simulink model "working_4states2"  (R2022b)
settings: Solver=FixedStepAuto  StartTime=0.0  StopTime=10.0  FixedStep=1e-3  RelTol=1e-3  EnableMultiTasking=on
undefined symbols (not defined in the file): a, A0, A1, b, c, D0, D1, D10, D11, D12, D13, D2, D3, D4, D5, D6, D7, D8, D9, PTA0, PTA1, PTA2, PTB2, PTB23, PTB3, PTB9, PTC16, PTC17, PTC2, PTC3, PTC4, PTD0, PTD1, PTD2, PTD3
libraries: frdmk64flib x22, etargetslib x2, dspstat3 x1, hdlsllib x1
settings Model: ExtModeTrigDuration=5  Creator=qasim  LastModifiedBy=Venka
settings SolverCC: AlgebraicLoopSolver=TrustRegion
settings OptimizationCC: EnhancedBackFolding=on  PassReuseOutputArgsAs=Individual arguments  ZeroExternalMemoryAtStartup=off  ZeroInternalMemoryAtStartup=off  MaxStackSize=64  OptimizeBlockOrder=speed  DifferentSizesBufferReuse=on  OptimizationCustomize=off  EfficientTunableParamExpr=on
settings DebuggingCC: ParameterTunabilityLossMsg=error  UnconnectedInputMsg=warning  UnconnectedOutputMsg=warning  UnconnectedLineMsg=warning  SFMachineParentedDataDiag=warning
settings HardwareCC: ProdBitPerPointer=32  ProdBitPerSizeT=32  ProdBitPerPtrDiffT=32  ProdLargestAtomicInteger=Long  ProdLargestAtomicFloat=Double  ProdWordSize=32  ProdHWDeviceType=ARM Compatible->ARM Cortex
settings ModelReferenceCC: EnableRefExpFcnMdlSchedulingChecks=on
settings SFSimCC: MATLABDynamicMemAlloc=off
settings RTWCC: Description=Embedded Coder  SystemTargetFile=ert.tlc  HardwareBoard=NXP FRDM-K64F  TLCOptions="-aInlineSetEventsForThisBaseRateFcn=TLC_FALSE -aSuppressMultiTaskScheduler=TLC_FALSE  -aRateBasedStepFcn=0"  TemplateMakefile=ert_default_tmf  Toolchain=GNU Tools for ARM Embedded Processors
settings CodeAppCC: ForceParamTrailComments=on  IgnoreCustomStorageClasses=off  OperatorAnnotations=on  SimulinkDataObjDesc=on  SFDataObjDesc=on  InsertBlockDesc=on

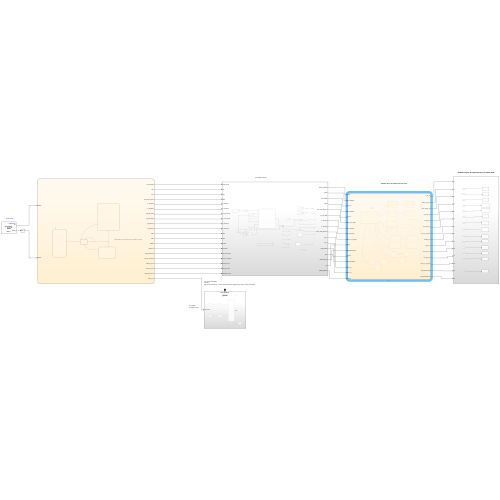
[thumbnail: Simulink's stored preview of the top-level diagram]
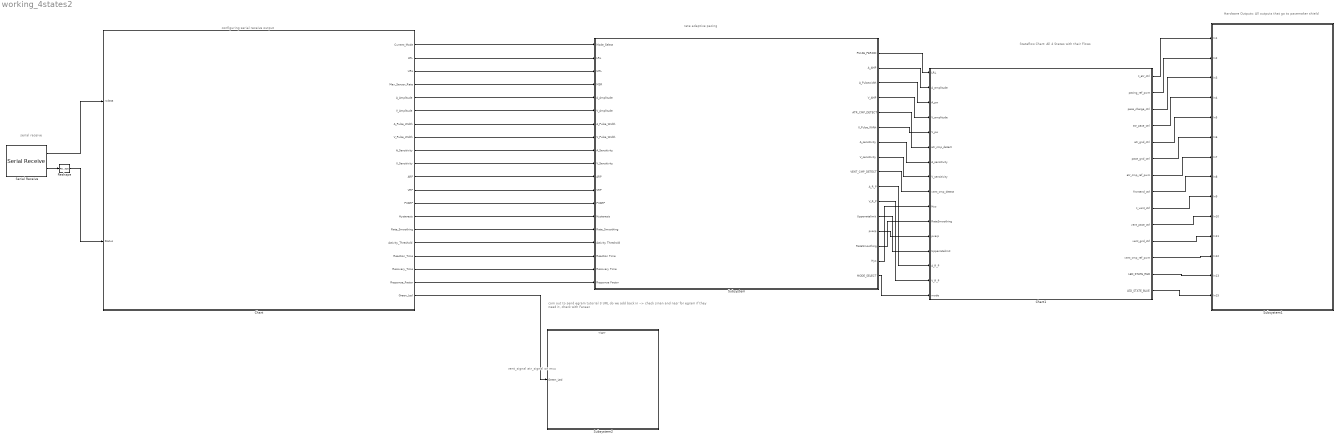
== system working_4states2 ==
  note: vent_signal
      | atr_signal on mcu
  note: rate adaptive pacing
  note: com out to send egram
      | tutorial 3
      | URL do we add back in --> check sinan and nasr for egram if they need it, check with Faraaz
  note: configuring serial receive output
  note: serial receive
  note: Stateflow Chart: All 4 States with their Flows
  note: Hardware Outputs: All outputs that go to pacemaker shield
  Chart : Stateflow chart  TreatAsAtomicUnit=on
      settings: PortSchema="{\"entries\":[{\"content\":{\"sides\":[{\"content\":{\"connectorIds\":[\"In1\",\"In2\"]},\"type\":\"ConnectorPlacement.EquallySpacedRectSide\",\"uuid\":\"8252b096-ee07-43c1-a389-abcea636169e\"},{\"content\":{\"connectorIds\":[\"Out12\",\"Out1\",\"Out16\",\"Out6\",\"Out8\",\"Out18\",\"Out10\",\"Out2\",\"Out11\",\"Out19\",\"Out9\",\"Out17\",\"Out14\",\"Out13\",\"Out15\",\"Out7\",\"Out5\",\"Out4\",\"Out3\",\"Out20\"],\"side\":\"RIGHT\"},\"type\":\"ConnectorPlacement.EquallySpacedRectSide\",\"uuid\":\"6509d00a-23de-4c51-a2fd-aafeb9bf7496\"},{\"content\":{\"connectorIds\":[],\"side\":\"TOP\"},\"type\":\"ConnectorPlacement.EquallySpacedRectSide\",\"uuid\":\"7ce604d1-90fd-4e3f-a76f-dae8bfc557ef\"}]},\"type\":\"ConnectorPlacement.EquallySpacedConnector\",\"uuid\":\"aa5568fb-1845-4bf2-8442-67645cd91be1\"}],\"packageUris\":[\"http://schema.mathworks.com/mf0/Connector/19700101\"],\"version\":\"1.0\"}"
  Chart1 : Stateflow chart  TreatAsAtomicUnit=on
      settings: PortSchema="{\"entries\":[{\"content\":{\"sides\":[{\"content\":{\"connectorIds\":[\"In1\",\"In4\",\"In5\",\"In9\",\"In10\",\"In2\",\"In7\",\"In8\",\"In6\",\"In11\",\"In12\",\"In13\",\"In14\",\"In15\",\"In16\",\"In3\"]},\"type\":\"ConnectorPlacement.EquallySpacedRectSide\",\"uuid\":\"9ebc7a7a-d83d-48fa-a96d-77ac692b9900\"},{\"content\":{\"connectorIds\":[\"Out1\",\"Out2\",\"Out3\",\"Out4\",\"Out5\",\"Out6\",\"Out7\",\"Out8\",\"Out9\",\"Out10\",\"Out11\",\"Out12\",\"Out13\",\"Out14\"],\"side\":\"RIGHT\"},\"type\":\"ConnectorPlacement.EquallySpacedRectSide\",\"uuid\":\"b238fc19-89ba-47ab-b52b-92ee760fd465\"},{\"content\":{\"connectorIds\":[],\"side\":\"TOP\"},\"type\":\"ConnectorPlacement.EquallySpacedRectSide\",\"uuid\":\"260cfadc-f762-444a-84c6-2a5806da8ce4\"}]},\"type\":\"ConnectorPlacement.EquallySpacedConnector\",\"uuid\":\"de40cf96-4d97-4a60-8c1b-853002d7031e\"}],\"packageUris\":[\"http://schema.mathworks.com/mf0/Connector/19700101\"],\"version\":\"1.0\"}"
  Reshape : Reshape
  Serial Receive : frdmk64flib/Serial Receive  SCIModule=0  Baudrate=uint32(9600)  Parity=None  StopBits=1  HardwareFlowControl=None  ByteOrder=LittleEndian  DataType=uint8  DataLength=52  BlockingMode=off  OutputStatus=on  SampleTime=-1
  Subsystem : Subsystem
  Subsystem1 : Subsystem
  Subsystem2 : Subsystem
  wires:
  Chart1/7(atr_cmp_ref_pwm) -> Subsystem1/7(In7)
  Chart1/5(atr_gnd_ctrl) -> Subsystem1/5(In5)
  Chart1/2(pacing_ref_pwm) -> Subsystem1/2(In2)
  Chart1/8(frontend_ctrl) -> Subsystem1/8(In8)
  Chart1/13(LED_STATE_RED) -> Subsystem1/13(In13)
  Chart1/3(pace_charge_ctrl) -> Subsystem1/3(In3)
  Chart1/11(vent_gnd_ctrl) -> Subsystem1/11(In11)
  Chart1/4(atr_pace_ctrl) -> Subsystem1/4(In4)
  Chart1/12(vent_cmp_ref_pwm) -> Subsystem1/12(In12)
  Chart1/9(z_vent_ctrl) -> Subsystem1/9(In9)
  Chart1/14(LED_STATE_BLUE) -> Subsystem1/14(In15)
  Chart1/1(z_atr_ctrl) -> Subsystem1/1(In1)
  Chart1/10(vent_pace_ctrl) -> Subsystem1/10(In10)
  Chart1/6(pace_gnd_ctrl) -> Subsystem1/6(In6)
  Subsystem/5(ATR_CMP_DETECT) -> Chart1/2(atr_cmp_detect)
  Subsystem/9(VENT_CMP_DETECT) -> Chart1/6(vent_cmp_detect)
  Subsystem/16(MODE_SELECT) -> Chart1/3(mode)
  Subsystem/2(A_AMP) -> Chart1/4(A_amplitude)
  Subsystem/3(A_Pulsewidth) -> Chart1/5(A_pw)
  Subsystem/1(PULSE_PERIOD) -> Chart1/1(LRL)
  Serial Receive/1 -> Chart/1(rxdata)
  Chart/1(LRL) -> Subsystem/2(LRL)
  Chart/6(Max_Sensor_Rate) -> Subsystem/4(MSR)
  Chart/7(Activity_Threshold) -> Subsystem/16(Activity Threshold)
  Chart/3(Response_Factor) -> Subsystem/19(Response Factor)
  Chart/5(Reaction_Time) -> Subsystem/17(Reaction Time)
  Chart/4(Recovery_Time) -> Subsystem/18(Recovery Time)
  Chart/8(A_Amplitude) -> Subsystem/5(A_Amplitude)
  Chart/11(A_Sensitivity) -> Subsystem/9(A_Sensitivity)
  Chart/19(V_Sensitivity) -> Subsystem/10(V_Sensitivity)
  Chart/18(V_Amplitude) -> Subsystem/6(V_Amplitude)
  Chart/10(A_Pulse_Width) -> Subsystem/7(A_Pulse_Width)
  Chart/2(V_Pulse_Width) -> Subsystem/8(V_Pulse_Width)
  Chart/9(ARP) -> Subsystem/11(ARP)
  Chart/12(Current_Mode) -> Subsystem/1(Mode_Select)
  Chart/13(Hysteresis) -> Subsystem/14(Hysteresis)
  Chart/17(VRP) -> Subsystem/12(VRP)
  Chart/16(URL) -> Subsystem/3(URL)
  Chart/14(PVARP) -> Subsystem/13(PVARP)
  Chart/15(Rate_Smoothing) -> Subsystem/15(Rate_Smoothing)
  Subsystem/4(V_AMP) -> Chart1/9(V_amplitude)
  Subsystem/6(V_Pulse_Wifth) -> Chart1/10(V_pw)
  Subsystem/7(A_sensitivity) -> Chart1/7(A_sensitivity)
  Subsystem/8(V_sensitivity) -> Chart1/8(V_sensitivity)
  Subsystem/15(Hys) -> Chart1/11(Hys)
  Subsystem/14(RateSmoothing) -> Chart1/12(RateSmoothing)
  Subsystem/13(pvarp) -> Chart1/13(pvarp)
  Subsystem/12(Upperratelimit) -> Chart1/14(Upperratelimit)
  Subsystem/11(V_R_P) -> Chart1/16(V_R_P)
  Subsystem/10(A_R_P) -> Chart1/15(A_R_P)
  Serial Receive/2 -> Reshape/1
  Reshape/1 -> Chart/2(Status)
  Chart/20(Green_Led) -> Subsystem2/1(Green_Led)

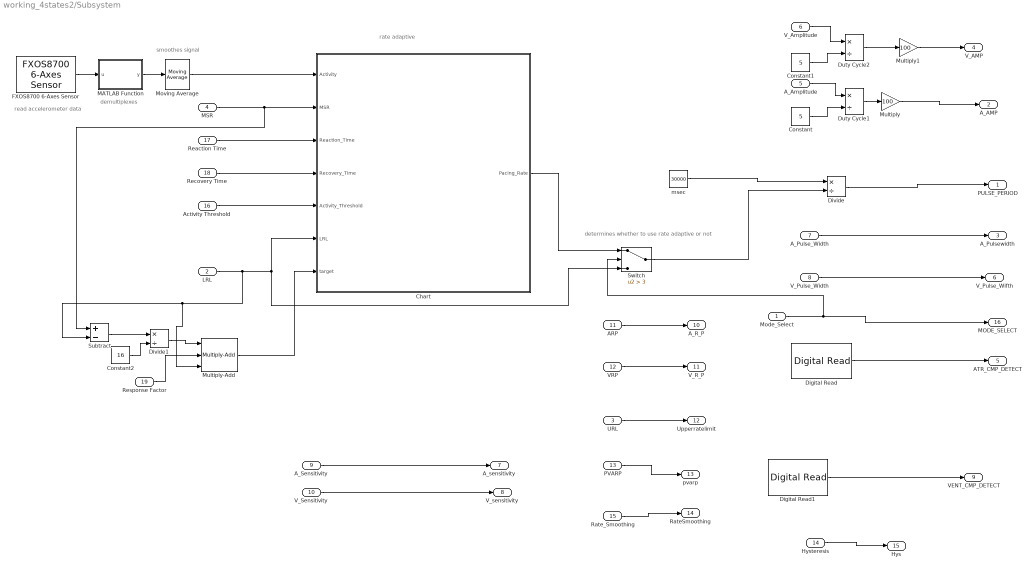
== system working_4states2/Subsystem ==
  note: rate adaptive
  note: determines whether to use rate adaptive or not
  note: smoothes signal
  note: demultiplexes
  note: read accelerometer data
  Mode_Select : Inport
  LRL : Inport  Port=2
  URL : Inport  Port=3
  MSR : Inport  Port=4
  A_Amplitude : Inport  Port=5
  V_Amplitude : Inport  Port=6
  A_Pulse_Width : Inport  Port=7
  V_Pulse_Width : Inport  Port=8
  A_Sensitivity : Inport  Port=9
  V_Sensitivity : Inport  Port=10
  ARP : Inport  Port=11
  VRP : Inport  Port=12
  PVARP : Inport  Port=13
  Hysteresis : Inport  Port=14
  Rate_Smoothing : Inport  Port=15
  Activity Threshold : Inport  Port=16
  Reaction Time : Inport  Port=17
  Recovery Time : Inport  Port=18
  Response Factor : Inport  Port=19
  Chart : Stateflow chart  TreatAsAtomicUnit=on
  Constant : Constant  Value=5
  Constant1 : Constant  Value=5
  Constant2 : Constant  Value=16
  Digital Read : frdmk64flib/Digital Read  Whichpin=PTC16 (D0)  SampleTime=-1
  Digital Read1 : frdmk64flib/Digital Read  Whichpin=PTC17 (D1)  SampleTime=-1
  Divide : Product  Inputs=*/
  Divide1 : Product  Inputs=*/
  Duty Cycle1 : Product  Inputs=*/
  Duty Cycle2 : Product  Inputs=*/
  FXOS8700 6-Axes Sensor : frdmk64flib/FXOS8700 6-Axes Sensor  Activesensor=Accelerometer only  ODR=100Hz  HybridODR=400Hz  Accelfullrange=-4g to +4g  SampleTime=-1
  MATLAB Function : MATLAB Function  TreatAsAtomicUnit=on
  Moving Average : dspstat3/Moving Average  Method=Sliding window  ForgettingFactorPort=off  SpecifyWindowLength=on  WindowLength=500  OverlapLength=499  AllowArbitraryInputLength=off  ForgettingFactor=0.9  SimulateUsing=Code generation
  Multiply : Gain  Gain=100
  Multiply-Add : hdlsllib/HDL Operations/Multiply-Add  Function=c+(a.*b)  datatype=Inherit: Inherit via internal rule  DoSatur=off  FMA=off
  Multiply1 : Gain  Gain=100
  Subtract : Sum  Inputs=+-
  Switch : Switch  Criteria=u2 > Threshold  Threshold=3  SaturateOnIntegerOverflow=off  InputSameDT=off
  msec : Constant  Value=30000
  PULSE_PERIOD : Outport
  A_AMP : Outport  Port=2
  A_Pulsewidth : Outport  Port=3
  V_AMP : Outport  Port=4
  ATR_CMP_DETECT : Outport  Port=5
  V_Pulse_Wifth : Outport  Port=6
  A_sensitivity : Outport  Port=7
  V_sensitivity : Outport  Port=8
  VENT_CMP_DETECT : Outport  Port=9
  A_R_P : Outport  Port=10
  V_R_P : Outport  Port=11
  Upperratelimit : Outport  Port=12
  pvarp : Outport  Port=13
  RateSmoothing : Outport  Port=14
  Hys : Outport  Port=15
  MODE_SELECT : Outport  Port=16
  wires:
  Moving Average/1 -> Chart/1(Activity)
  LRL/1 -> Multiply-Add/3, Subtract/2, Switch/3, Chart/6(LRL)
  Response Factor/1 -> Multiply-Add/2
  FXOS8700 6-Axes Sensor/1 -> MATLAB Function/1(u)
  Activity Threshold/1 -> Chart/5(Activity_Threshold)
  MSR/1 -> Subtract/1, Chart/2(MSR)
  Reaction Time/1 -> Chart/3(Reaction_Time)
  MATLAB Function/1(y) -> Moving Average/1
  Chart/1(Pacing_Rate) -> Switch/1
  Recovery Time/1 -> Chart/4(Recovery_Time)
  Multiply/1 -> A_AMP/1
  A_Amplitude/1 -> Duty Cycle1/1
  Duty Cycle1/1 -> Multiply/1
  Divide/1 -> PULSE_PERIOD/1
  Mode_Select/1 -> Switch/2, MODE_SELECT/1
  Constant/1 -> Duty Cycle1/2
  msec/1 -> Divide/1
  Digital Read/1 -> ATR_CMP_DETECT/1
  Digital Read1/1 -> VENT_CMP_DETECT/1
  Constant1/1 -> Duty Cycle2/2
  V_Amplitude/1 -> Duty Cycle2/1
  Duty Cycle2/1 -> Multiply1/1
  Multiply1/1 -> V_AMP/1
  ARP/1 -> A_R_P/1
  VRP/1 -> V_R_P/1
  URL/1 -> Upperratelimit/1
  PVARP/1 -> pvarp/1
  Rate_Smoothing/1 -> RateSmoothing/1
  Hysteresis/1 -> Hys/1
  Subtract/1 -> Divide1/1
  Divide1/1 -> Multiply-Add/1
  Constant2/1 -> Divide1/2
  Multiply-Add/1 -> Chart/7(target)
  A_Sensitivity/1 -> A_sensitivity/1
  V_Sensitivity/1 -> V_sensitivity/1
  Switch/1 -> Divide/2
  A_Pulse_Width/1 -> A_Pulsewidth/1
  V_Pulse_Width/1 -> V_Pulse_Wifth/1

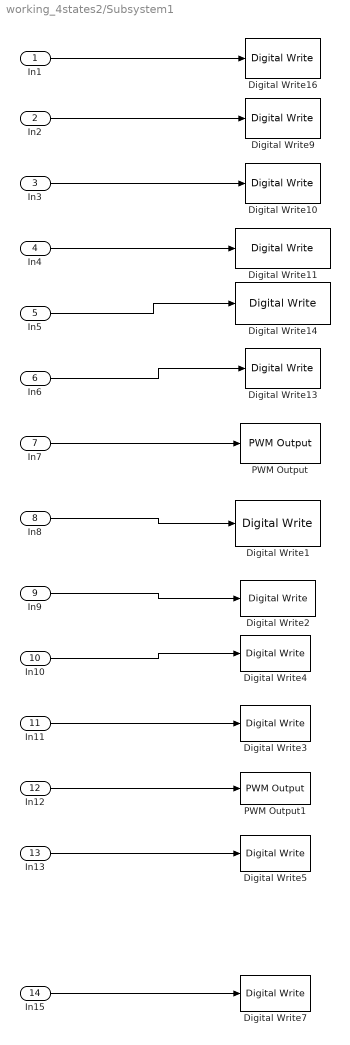
== system working_4states2/Subsystem1 ==
  In1 : Inport
  In2 : Inport  Port=2
  In3 : Inport  Port=3
  In4 : Inport  Port=4
  In5 : Inport  Port=5
  In6 : Inport  Port=6
  In7 : Inport  Port=7
  In8 : Inport  Port=8
  In9 : Inport  Port=9
  In10 : Inport  Port=10
  In11 : Inport  Port=11
  In12 : Inport  Port=12
  In13 : Inport  Port=13
  In15 : Inport  Port=14
  Digital Write1 : frdmk64flib/Digital Write  Whichpin=PTD1 (D13)
  Digital Write10 : frdmk64flib/Digital Write  Whichpin=PTB9 (D2)
  Digital Write11 : frdmk64flib/Digital Write  Whichpin=PTA0 (D8)
  Digital Write13 : frdmk64flib/Digital Write  Whichpin=PTD0 (D10)
  Digital Write14 : frdmk64flib/Digital Write  Whichpin=PTD2 (D11)
  Digital Write16 : frdmk64flib/Digital Write  Whichpin=PTB23 (D4)
  Digital Write2 : frdmk64flib/Digital Write  Whichpin=PTC3 (D7)
  Digital Write3 : frdmk64flib/Digital Write  Whichpin=PTD3 (D12)
  Digital Write4 : frdmk64flib/Digital Write  Whichpin=PTC4 (D9)
  Digital Write5 : frdmk64flib/Digital Write  Whichpin=RED_LED
  Digital Write7 : frdmk64flib/Digital Write  Whichpin=BLUE_LED
  Digital Write9 : frdmk64flib/Digital Write  Whichpin=PTA2 (D5)
  PWM Output : frdmk64flib/PWM Output  Whichpin=PTC2 (D6)  InitialFrequency=2000  InitialDutyCycle=0
  PWM Output1 : frdmk64flib/PWM Output  Whichpin=PTA1 (D3)  InitialFrequency=2000  InitialDutyCycle=0
  wires:
  In1/1 -> Digital Write16/1
  In2/1 -> Digital Write9/1
  In3/1 -> Digital Write10/1
  In4/1 -> Digital Write11/1
  In5/1 -> Digital Write14/1
  In6/1 -> Digital Write13/1
  In7/1 -> PWM Output/1
  In8/1 -> Digital Write1/1
  In9/1 -> Digital Write2/1
  In10/1 -> Digital Write4/1
  In11/1 -> Digital Write3/1
  In12/1 -> PWM Output1/1
  In13/1 -> Digital Write5/1
  In15/1 -> Digital Write7/1

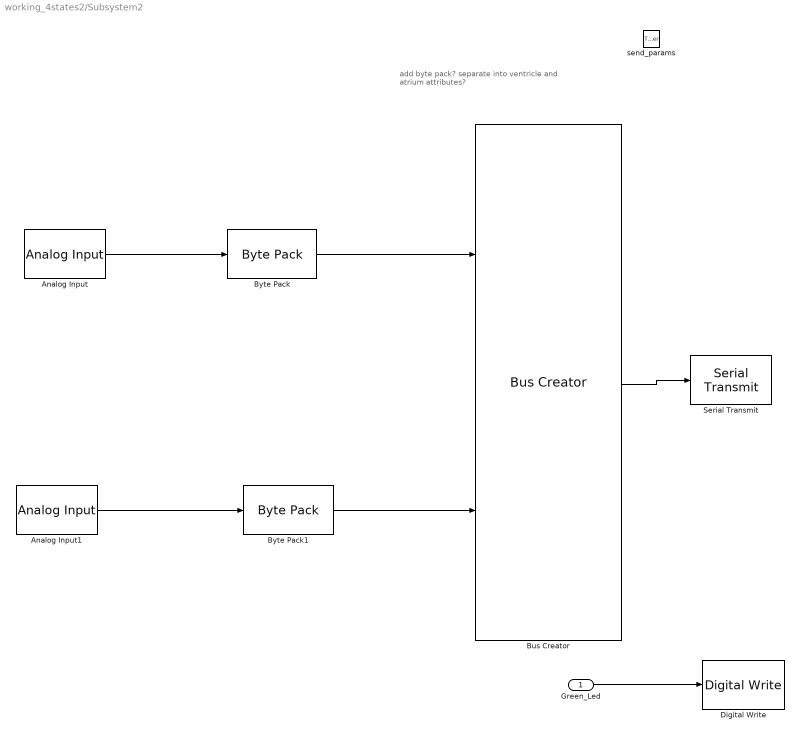
== system working_4states2/Subsystem2 ==
  note: add byte pack?
      | separate into ventricle and atrium attributes?
  Green_Led : Inport
  send_params : TriggerPort  TriggerType=function-call  IsSimulinkFunction=on  FunctionName=send_params  VariantControl=Variant  PortDimensions=1
  Analog Input : frdmk64flib/Analog Input  Whichpin=PTB2 (A0)  SampleTime=-1
  Analog Input1 : frdmk64flib/Analog Input  Whichpin=PTB3 (A1)  SampleTime=-1
  Bus Creator : BusCreator  Inputs=2
  Byte Pack : etargetslib/Byte Pack  datatypes={'double'}  byteAlign=1
  Byte Pack1 : etargetslib/Byte Pack  datatypes={'double'}  byteAlign=1
  Digital Write : frdmk64flib/Digital Write  Whichpin=GREEN_LED
  Serial Transmit : frdmk64flib/Serial Transmit  SCIModule=0  Baudrate=uint32(9600)  Parity=None  StopBits=1  HardwareFlowControl=None  ByteOrder=LittleEndian  BlockingMode=on  OutputStatus=off
  wires:
  Bus Creator/1 -> Serial Transmit/1
  Analog Input/1 -> Byte Pack/1
  Analog Input1/1 -> Byte Pack1/1
  Byte Pack/1 -> Bus Creator/1
  Byte Pack1/1 -> Bus Creator/2
  Green_Led/1 -> Digital Write/1

== stateflow chart working_4states2/Chart1 ==
  state charging
    entry:
    %charging C22
    %discharging C21
    atr_pace_ctrl = 0; %do not want c22 to discharge
    pacing_ref_pwm = A_amplitude; %send in signal
    pace_charge_ctrl = 1;
    pace_gnd_ctrl = 0; %discharges C21
    atr_gnd_ctrl = 1; %1 when discharging through atrium
    atr_cmp_ref_pwm = 1; %send in threshold signal, if heart is less then we will send signal
    %average threshold amplitude is 80
    z_atr_ctrl = 0; %connects impedance circuit to atrium ring electrode output is at z_signal pin
    LED_STATE_RED = 0;
    LED_STATE_BLUE = 1;
  state pacing
    entry:
    %charging C21
    %discharging C22
    atr_gnd_ctrl = 0;
    atr_pace_ctrl = 1;
    z_atr_ctrl = 0;
    pace_charge_ctrl = 0;
    pace_gnd_ctrl = 1;
    atr_gnd_ctrl = 0;
    pacing_ref_pwm = A_amplitude;
    LED_STATE_RED = 1;
    LED_STATE_BLUE = 0;
  note: AOO
  note: LIST OF MODES
      |
      | mode 1 = AOO
      | mode 2 = VOO
      | mode 3 = AAI
      | mode 4 = VVI
  note: Initializes all variables that will be used for charging and pacing modes
  state pacing1
    entry:
    %charging C21
    %discharging C22
    vent_gnd_ctrl = 0;
    vent_pace_ctrl = 1;
    z_vent_ctrl = 0;
    pace_charge_ctrl = 0;
    pace_gnd_ctrl = 1;
    vent_gnd_ctrl = 0;
    pacing_ref_pwm = V_amplitude;
    LED_STATE_RED=1;
    %LED_STATE_GREEN=0;
  state charging1
    entry:
    %charging C22
    %discharging C21
    vent_pace_ctrl = 0; %do not want c22 to discharge
    pacing_ref_pwm = V_amplitude; %send in signal
    pace_charge_ctrl = 1;
    pace_gnd_ctrl = 0; %discharges C21
    vent_gnd_ctrl = 1; %1 when discharging through VENT
    vent_cmp_ref_pwm = 80; %send in threshold signal, if heart is less then we will send signal
    %average threshold amplitude is 80
    z_vent_ctrl = 0; %connects impedance circuit to atrium ring electrode output is at z_signal pin
    LED_STATE_RED=0;
    %LED_STATE_GREEN=1;
  note: start_here
  state INIT
    entry:
    z_vent_ctrl = 0;
    z_atr_ctrl = 0;
    pace_charge_ctrl=0;
    vent_pace_ctrl = 0;
    atr_pace_ctrl = 0;
    atr_gnd_ctrl = 0;
    vent_gnd_ctrl = 0;
    pace_gnd_ctrl = 0;
    frontend_ctrl = 1;
    atr_cmp_ref_pwm = 50;
    vent_cmp_ref_pwm = 50;
    %LRL is what tells you when to send in a pulse if
    %incoming rate is lower than LRL
  note: VOO
  state pacing2
    entry:
    %charging C21
    %discharging C22
    atr_gnd_ctrl = 0;
    atr_pace_ctrl = 1;
    z_atr_ctrl = 0;
    pace_charge_ctrl = 0;
    pace_gnd_ctrl = 1;
    pacing_ref_pwm = A_amplitude;
    frontend_ctrl = 0;
    LED_STATE_RED = 0;
    LED_STATE_BLUE = 1;
  note: AAI
  state charging2
    entry:
    %CHARGING
    %charging C22
    %discharging C21
    atr_pace_ctrl = 0; %do not want c22 to discharge
    pacing_ref_pwm = A_amplitude; %send in signal
    pace_charge_ctrl = 1;
    pace_gnd_ctrl = 0; %discharges C21
    atr_gnd_ctrl = 1; %1 when discharging through atr
    %average threshold amplitude is 80
    z_atr_ctrl = 0; %connects impedance circuit to atrium ring electrode output is at z_signal pin
    %SENSING
    frontend_ctrl = 1;
    atr_cmp_ref_pwm = 50; %send in threshold signal, if heart is less then we will send signal
    LED_STATE_RED = 1;
    LED_STATE_BLUE = 0;
  state charging3
    entry:
    %CHARGING
    %charging C22
    %discharging C21
    vent_pace_ctrl = 0; %do not want c22 to discharge
    pacing_ref_pwm = V_amplitude; %send in signal
    pace_charge_ctrl = 1;
    pace_gnd_ctrl = 0; %discharges C21
    vent_gnd_ctrl = 1; %1 when discharging through vent
    %average threshold amplitude is 80
    z_vent_ctrl = 0; %connects impedance circuit to vent ring electrode output is at z_signal pin
    %SENSING
    frontend_ctrl = 1;
    vent_cmp_ref_pwm = 50; %send in threshold signal, if heart is less then we will send signal
    LED_STATE_RED=1;
    %LED_STATE_GREEN=0
  state pacing3
    entry:
    %charging C21
    %discharging C22
    vent_gnd_ctrl = 0;
    vent_pace_ctrl = 1;
    z_vent_ctrl = 0;
    pace_charge_ctrl = 0;
    pace_gnd_ctrl = 1;
    pacing_ref_pwm = V_amplitude;
    frontend_ctrl = 0;
    LED_STATE_RED=0;
    %LED_STATE_GREEN=1;
  note: AOOr
  state charging5
    entry:
    %charging C22
    %discharging C21
    atr_pace_ctrl = 0; %do not want c22 to discharge
    pacing_ref_pwm = A_amplitude; %send in signal
    pace_charge_ctrl = 1;
    pace_gnd_ctrl = 0; %discharges C21
    atr_gnd_ctrl = 1; %1 when discharging through atrium
    atr_cmp_ref_pwm = 80; %send in threshold signal, if heart is less then we will send signal
    %average threshold amplitude is 80
    z_atr_ctrl = 0; %connects impedance circuit to atrium ring electrode output is at z_signal pin
  state pacing4
    entry:
    %charging C21
    %discharging C22
    atr_gnd_ctrl = 0;
    atr_pace_ctrl = 1;
    z_atr_ctrl = 0;
    pace_charge_ctrl = 0;
    pace_gnd_ctrl = 1;
    atr_gnd_ctrl = 0;
    pacing_ref_pwm = A_amplitude;
  note: VVI
  note: VOOR
  state charging4
    entry:
    %charging C22
    %discharging C21
    vent_pace_ctrl = 0; %do not want c22 to discharge
    pacing_ref_pwm = V_amplitude; %send in signal
    pace_charge_ctrl = 1;
    pace_gnd_ctrl = 0; %discharges C21
    vent_gnd_ctrl = 1; %1 when discharging through VENT
    vent_cmp_ref_pwm = 80; %send in threshold signal, if heart is less then we will send signal
    %average threshold amplitude is 80
    z_vent_ctrl = 0; %connects impedance circuit to atrium ring electrode output is at z_signal pin
    LED_STATE_RED=0;
    %LED_STATE_GREEN=1;
  state pacing7
    entry:
    %charging C21
    %discharging C22
    vent_gnd_ctrl = 0;
    vent_pace_ctrl = 1;
    z_vent_ctrl = 0;
    pace_charge_ctrl = 0;
    pace_gnd_ctrl = 1;
    vent_gnd_ctrl = 0;
    pacing_ref_pwm = V_amplitude;
    LED_STATE_RED=1;
    %LED_STATE_GREEN=0;
  note: AAIR
  state discharging
    during:
    pace_charge_ctrl = 0;
    pace_gnd_ctrl = 1;
    atr_pace_ctrl = 1;
    atr_gnd_ctrl = 0;
    z_atr_ctrl = 0;
    z_vent_ctrl = 0;
    vent_gnd_ctrl = 0;
    vent_pace_ctrl = 0;
  state charging6
    during:
    %CHARGING
    %charging C22
    %discharging C21
    pacing_ref_pwm = A_amplitude; %send in signal
    atr_pace_ctrl = 0;
    vent_pace_ctrl = 0;
    pace_charge_ctrl = 1;
    pace_gnd_ctrl = 1;
    vent_pace_ctrl = 0;
    z_atr_ctrl = 0;
    z_vent_ctrl = 0;
    atr_pace_ctrl = 0;
    atr_gnd_ctrl = 1;
    vent_gnd_ctrl = 0;
  state choosing
    during:
    pace_gnd_ctrl = 1;
    vent_pace_ctrl  = 0;
    z_atr_ctrl  = 0;
    z_vent_ctrl  = 0;
    atr_pace_ctrl  = 0;
    atr_gnd_ctrl  = 1;
    vent_gnd_ctrl = 0;
    atr_pace_ctrl  = 0;
    vent_pace_ctrl  = 0;
    pacing_ref_pwm = A_amplitude;
    pace_charge_ctrl = 1;
    frontend_ctrl = 1;
  note: VVIR
  state charging7
    during:
    %CHARGING
    %charging C22
    %discharging C21
    pacing_ref_pwm = V_amplitude; %send in signal
    atr_pace_ctrl = 0;
    vent_pace_ctrl = 0;
    pace_charge_ctrl = 1;
    pace_gnd_ctrl = 1;
    vent_pace_ctrl = 0;
    z_atr_ctrl = 0;
    z_vent_ctrl = 0;
    atr_pace_ctrl = 0;
    atr_gnd_ctrl = 0;
    vent_gnd_ctrl = 1;
  state discharging1
    during:
    pace_charge_ctrl = 0;
    pace_gnd_ctrl = 1;
    atr_pace_ctrl = 0;
    atr_gnd_ctrl = 0;
    z_atr_ctrl = 0;
    z_vent_ctrl = 0;
    vent_gnd_ctrl = 0;
    vent_pace_ctrl = 1;
  state choosing1
    during:
    pace_gnd_ctrl = 1;
    vent_pace_ctrl  = 0;
    z_atr_ctrl  = 0;
    z_vent_ctrl  = 0;
    atr_pace_ctrl  = 0;
    atr_gnd_ctrl  = 0;
    vent_gnd_ctrl = 1;
    atr_pace_ctrl  = 0;
    vent_pace_ctrl  = 0;
    pacing_ref_pwm = V_amplitude;
    pace_charge_ctrl = 1;
  charging -> pacing [order 1] : [after(LRL - A_pw, msec)]
  INIT -> charging [order 1] : [mode ==0 ]
  pacing -> charging : [after(A_pw, msec)]
  charging -> INIT [order 2] : [mode ~= 0 ]
  INIT -> charging1 [order 2] : [mode == 1 ]
  (default) -> INIT
  charging1 -> pacing1 [order 1] : [after(LRL - V_pw, msec)]
  charging1 -> INIT [order 2] : [mode ~=1 ]
  pacing1 -> charging1 : [after(V_pw, msec)]
  (junction 118) -> charging2 [order 2] : [atr_cmp_detect == 1]
  charging2 -> INIT [order 2] : [mode ~=2 ]
  INIT -> INIT [order 5] : [mode ~= 0 | mode ~= 1 | mode ~= 2 | mode ~= 3| mode ~= 4 | mode ~= 5 | mode ~= 6 | mode ~= 7]
  INIT -> charging2 [order 3] : [mode ==2 ]
  charging2 -> (junction 118) [order 1]
  (junction 118) -> pacing2 [order 1] : after(LRL-A_pw, msec)[atr_cmp_detect==0]
  charging3 -> INIT [order 2] : [mode ~=3 ]
  INIT -> charging3 [order 4] : [mode == 3 ]
  charging7 -> INIT [order 3] : [mode ~= 7]
  INIT -> charging7 [order 9] : [mode == 7]
  charging6 -> INIT [order 3] : [mode ~= 6]
  charging4 -> INIT [order 2] : [mode ~= 5]
  INIT -> charging6 [order 8] : [mode == 6  ]
  INIT -> charging5 [order 6] : [mode ==4]
  INIT -> charging4 [order 7] : [mode == 5]
  charging5 -> INIT [order 2] : [mode ~= 4]
  pacing2 -> charging2 : [after(A_pw, msec)]
  (junction 122) -> charging3 [order 1] : [vent_cmp_detect == 1]
  charging3 -> (junction 122) [order 1]
  (junction 122) -> pacing3 [order 2] : after(LRL-V_pw, msec)[vent_cmp_detect==0]
  pacing3 -> charging3 : [after(V_pw, msec)]
  charging5 -> pacing4 [order 1] : [after(LRL - A_pw, msec)]
  pacing4 -> charging5 : [after(A_pw, msec)]
  charging4 -> pacing7 [order 1] : [after(LRL - V_pw, msec)]
  pacing7 -> charging4 : [after(V_pw, msec)]
  charging6 -> discharging [order 1] : after(LRL - A_pw - A_R_P, msec)
  charging6 -> (junction 208) [order 2] : [atr_cmp_detect == 1]
  (junction 208) -> choosing : after(LRL, msec)
  discharging -> choosing : after(A_pw, msec)
  choosing -> charging6 : after(A_R_P, msec)
  charging7 -> discharging1 [order 1] : after(LRL- V_pw - V_R_P, msec)
  charging7 -> (junction 217) [order 2] : [vent_cmp_detect == 1]
  (junction 217) -> choosing1 : after(LRL, msec)
  discharging1 -> choosing1 : after(V_pw, msec)
  choosing1 -> charging7 : after(V_R_P, msec)
  data: LRL input; z_atr_ctrl output; pacing_ref_pwm output; pace_charge_ctrl output; atr_pace_ctrl output; atr_gnd_ctrl output; pace_gnd_ctrl output; atr_cmp_ref_pwm output; atr_cmp_detect input; frontend_ctrl output; mode input; A_amplitude input; A_pw input; vent_cmp_detect input; A_sensitivity input; V_sensitivity input; z_vent_ctrl output; vent_pace_ctrl output; vent_gnd_ctrl output; vent_cmp_ref_pwm output; LED_STATE_RED output; LED_STATE_BLUE output; V_amplitude input; V_pw input; Hys input; RateSmoothing input; pvarp input; Upperratelimit input; A_R_P input; V_R_P input

== matlab function working_4states2/Subsystem/MATLAB Function ==
  data: u input; y output
function y = fcn(u)

y = sqrt(u(1)^2+u(2)^2+u(3)^2);

== stateflow chart working_4states2/Subsystem/Chart ==
  state Start
    entry:
    Pacing_Rate = LRL;
    Time = 0;
  state Increase_Rate
    entry:
    Time = 0;
    step_up = (target-LRL)/Reaction_Time;
    during:
    Pacing_Rate = Pacing_Rate + step_up;
    Time = Time + 1/1000;
    exit:
    Time = 0;
  state Decrease_Rate
    entry:
    Time = 0;
    step_down = (target-LRL)/Recovery_Time;
    during:
    Pacing_Rate = Pacing_Rate-step_down;
    Time = Time + 1/1000;
    exit:
    Time = 0;
  state Rate_below_LRL
    entry:
    Pacing_Rate = LRL;
  state Rate_above_LRL
    entry:
    Pacing_Rate = MSR;
  (default) -> Start
  Start -> Decrease_Rate [order 2] : [Activity > Activity_Threshold]
  Start -> Increase_Rate [order 1] : [Activity <= Activity_Threshold]
  Decrease_Rate -> Decrease_Rate [order 1] : [Time > Recovery_Time]{Time = 0}
  Increase_Rate -> Increase_Rate [order 1] : [Time > Reaction_Time]{Time = 0}
  Increase_Rate -> Decrease_Rate [order 2] : [Activity > Activity_Threshold]
  Decrease_Rate -> Increase_Rate [order 3] : [Activity <= Activity_Threshold]
  Decrease_Rate -> Rate_below_LRL [order 2] : [Pacing_Rate < LRL]
  Rate_below_LRL -> Decrease_Rate
  Increase_Rate -> Rate_above_LRL [order 3] : [Pacing_Rate >= MSR]
  Rate_above_LRL -> Increase_Rate
  data: Activity input; MSR input; Reaction_Time input; Recovery_Time input; Activity_Threshold input; LRL input; Pacing_Rate output; Time local; step_down local; step_up local; target input

== stateflow chart working_4states2/Chart ==
  state SET_PARAM
    entry:
    Current_Mode = cast(rxdata(3),'uint16');
    LRL=cast(rxdata(4),'uint16');
    URL=cast(rxdata(5),'uint16');
    Max_Sensor_Rate=cast(rxdata(6),'uint16');
    A_Amplitude = typecast(rxdata(7:14),'double');
    V_Amplitude = typecast(rxdata(15:22),'double');
    A_Pulse_Width = cast(rxdata(23),'uint16');
    V_Pulse_Width = cast(rxdata(24),'uint16');
    A_Sensitivity = typecast(rxdata(25:32),'double');
    V_Sensitivity = typecast(rxdata(33:40),'double');
    VRP = typecast(rxdata(41:42),'uint16');
    ARP = typecast(rxdata(43:44),'uint16');
    PVARP = typecast(rxdata(45:46),'uint16');
    Hysteresis = cast(rxdata(47),'uint16');
    Rate_Smoothing = cast(rxdata(48),'uint16');
    Activity_Threshold = cast(rxdata(49),'double');
    Reaction_Time = cast(rxdata(50),'uint16');
    Response_Factor = cast(rxdata(51),'uint16');
    Recovery_Time = cast(rxdata(52),'uint16');
    Green_Led = 1;
  note: Tutorial 3
  note: atrium and ventircular PWM and other shit
  state INITIAL
    entry:
    Current_Mode = 0;
    LRL=60;
    URL = 120;
    Max_Sensor_Rate=0;
    A_Amplitude=4;
    V_Amplitude = 4;
    A_Pulse_Width = 10;
    V_Pulse_Width=10;
    A_Sensitivity=4;
    V_Sensitivity=4;
    VRP =0;
    ARP =0;
    PVARP = 0;
    Rate_Smoothing = 0;
    Hysteresis = 0;
    Activity_Threshold=0.1;
    Reaction_Time=10;
    Response_Factor=10;
    Recovery_Time=10;
    Green_Led = 0;
  note: V_ = ventricular
      | volt = voltage
  state STANDBY
  note: DCM needs to have a byte that gives us transition information
  state ECHO_PARAM
    entry:
    send_params();
  SET_PARAM -> STANDBY
  (default) -> INITIAL
  (junction 10) -> SET_PARAM [order 1] : [rxdata(2) == hex2dec('55')]
  (junction 7) -> STANDBY [order 2]
  INITIAL -> STANDBY
  STANDBY -> (junction 7) : [Status(1) == 0]
  (junction 7) -> (junction 10) [order 1] : [rxdata(1) == hex2dec('16')]
  (junction 10) -> ECHO_PARAM [order 2] : [rxdata(2) == hex2dec('22')]
  ECHO_PARAM -> STANDBY
  data: rxdata input uint8; LRL output uint16; V_Pulse_Width output uint16; Response_Factor output uint16; Recovery_Time output uint16; Reaction_Time output uint16; Max_Sensor_Rate output uint16; Activity_Threshold output double; A_Amplitude output double; ARP output uint16; A_Pulse_Width output uint16; A_Sensitivity output double; Current_Mode output uint16; Hysteresis output uint16; PVARP output uint16; Rate_Smoothing output uint16; URL output uint16; VRP output uint16; V_Amplitude output double; V_Sensitivity output double; Status input uint8; Green_Led output
